simulink model "QueuingSys"  (R2019a)
settings: Solver=VariableStepAuto  StartTime=0.0  StopTime=100  RelTol=1e-3  EnableMultiTasking=on
undefined symbols (not defined in the file or in its folder): m, n
(part 5 of 5)

== matlab function QueuingSys/Distro/MMPPArrivalTime36/MMPP ==
  data: x input; T input; D input; x output; M input; T output; D output; t output; rn input; lambda output
function [x,T,D,t,lambda] = fcn(x,T,D,M,rn)
lambda = sum(M(x,:))-M(x,x);
trn = expinv(rn,lambda);
if trn > T(2)
    D =rand(2,1);
    T2 = expinv(D(2),lambda);
    j = 1;
    a = 0;
    b = sum(M(x,1:j));
    while ~(a < D(1) < b)
        j = j +1;
        a = sum(M(x,1:j));
        b = sum(M(x,1:j));
    end
    x = j;
    T(1) = T(2);
    T(2) = T2;
    lambda = sum(M(x,:))-M(x,x);
    trn = expinv(rn,lambda);
end
% x = j;
t = trn;% x(end);

== matlab function QueuingSys/Distro/MMPPArrivalTime37/MMPP ==
  data: x input; T input; D input; x output; M input; T output; D output; t output; rn input; lambda output
function [x,T,D,t,lambda] = fcn(x,T,D,M,rn)
lambda = sum(M(x,:))-M(x,x);
trn = expinv(rn,lambda);
if trn > T(2)
    D =rand(2,1);
    T2 = expinv(D(2),lambda);
    j = 1;
    a = 0;
    b = sum(M(x,1:j));
    while ~(a < D(1) < b)
        j = j +1;
        a = sum(M(x,1:j));
        b = sum(M(x,1:j));
    end
    x = j;
    T(1) = T(2);
    T(2) = T2;
    lambda = sum(M(x,:))-M(x,x);
    trn = expinv(rn,lambda);
end
% x = j;
t = trn;% x(end);

== matlab function QueuingSys/Distro/MMPPArrivalTime38/MMPP ==
  data: x input; T input; D input; x output; M input; T output; D output; t output; rn input; lambda output
function [x,T,D,t,lambda] = fcn(x,T,D,M,rn)
lambda = sum(M(x,:))-M(x,x);
trn = expinv(rn,lambda);
if trn > T(2)
    D =rand(2,1);
    T2 = expinv(D(2),lambda);
    j = 1;
    a = 0;
    b = sum(M(x,1:j));
    while ~(a < D(1) < b)
        j = j +1;
        a = sum(M(x,1:j));
        b = sum(M(x,1:j));
    end
    x = j;
    T(1) = T(2);
    T(2) = T2;
    lambda = sum(M(x,:))-M(x,x);
    trn = expinv(rn,lambda);
end
% x = j;
t = trn;% x(end);

== matlab function QueuingSys/Distro/MMPPArrivalTime39/MMPP ==
  data: x input; T input; D input; x output; M input; T output; D output; t output; rn input; lambda output
function [x,T,D,t,lambda] = fcn(x,T,D,M,rn)
lambda = sum(M(x,:))-M(x,x);
trn = expinv(rn,lambda);
if trn > T(2)
    D =rand(2,1);
    T2 = expinv(D(2),lambda);
    j = 1;
    a = 0;
    b = sum(M(x,1:j));
    while ~(a < D(1) < b)
        j = j +1;
        a = sum(M(x,1:j));
        b = sum(M(x,1:j));
    end
    x = j;
    T(1) = T(2);
    T(2) = T2;
    lambda = sum(M(x,:))-M(x,x);
    trn = expinv(rn,lambda);
end
% x = j;
t = trn;% x(end);

== matlab function QueuingSys/Distro/MMPPArrivalTime40/MMPP ==
  data: x input; T input; D input; x output; M input; T output; D output; t output; rn input; lambda output
function [x,T,D,t,lambda] = fcn(x,T,D,M,rn)
lambda = sum(M(x,:))-M(x,x);
trn = expinv(rn,lambda);
if trn > T(2)
    D =rand(2,1);
    T2 = expinv(D(2),lambda);
    j = 1;
    a = 0;
    b = sum(M(x,1:j));
    while ~(a < D(1) < b)
        j = j +1;
        a = sum(M(x,1:j));
        b = sum(M(x,1:j));
    end
    x = j;
    T(1) = T(2);
    T(2) = T2;
    lambda = sum(M(x,:))-M(x,x);
    trn = expinv(rn,lambda);
end
% x = j;
t = trn;% x(end);

== matlab function QueuingSys/Distro/MMPPArrivalTime41/MMPP ==
  data: x input; T input; D input; x output; M input; T output; D output; t output; rn input; lambda output
function [x,T,D,t,lambda] = fcn(x,T,D,M,rn)
lambda = sum(M(x,:))-M(x,x);
trn = expinv(rn,lambda);
if trn > T(2)
    D =rand(2,1);
    T2 = expinv(D(2),lambda);
    j = 1;
    a = 0;
    b = sum(M(x,1:j));
    while ~(a < D(1) < b)
        j = j +1;
        a = sum(M(x,1:j));
        b = sum(M(x,1:j));
    end
    x = j;
    T(1) = T(2);
    T(2) = T2;
    lambda = sum(M(x,:))-M(x,x);
    trn = expinv(rn,lambda);
end
% x = j;
t = trn;% x(end);

== matlab function QueuingSys/Distro/MMPPArrivalTime42/MMPP ==
  data: x input; T input; D input; x output; M input; T output; D output; t output; rn input; lambda output
function [x,T,D,t,lambda] = fcn(x,T,D,M,rn)
lambda = sum(M(x,:))-M(x,x);
trn = expinv(rn,lambda);
if trn > T(2)
    D =rand(2,1);
    T2 = expinv(D(2),lambda);
    j = 1;
    a = 0;
    b = sum(M(x,1:j));
    while ~(a < D(1) < b)
        j = j +1;
        a = sum(M(x,1:j));
        b = sum(M(x,1:j));
    end
    x = j;
    T(1) = T(2);
    T(2) = T2;
    lambda = sum(M(x,:))-M(x,x);
    trn = expinv(rn,lambda);
end
% x = j;
t = trn;% x(end);

== matlab function QueuingSys/Distro/MMPPArrivalTime43/MMPP ==
  data: x input; T input; D input; x output; M input; T output; D output; t output; rn input; lambda output
function [x,T,D,t,lambda] = fcn(x,T,D,M,rn)
lambda = sum(M(x,:))-M(x,x);
trn = expinv(rn,lambda);
if trn > T(2)
    D =rand(2,1);
    T2 = expinv(D(2),lambda);
    j = 1;
    a = 0;
    b = sum(M(x,1:j));
    while ~(a < D(1) < b)
        j = j +1;
        a = sum(M(x,1:j));
        b = sum(M(x,1:j));
    end
    x = j;
    T(1) = T(2);
    T(2) = T2;
    lambda = sum(M(x,:))-M(x,x);
    trn = expinv(rn,lambda);
end
% x = j;
t = trn;% x(end);

== matlab function QueuingSys/Distro/MMPPArrivalTime44/MMPP ==
  data: x input; T input; D input; x output; M input; T output; D output; t output; rn input; lambda output
function [x,T,D,t,lambda] = fcn(x,T,D,M,rn)
lambda = sum(M(x,:))-M(x,x);
trn = expinv(rn,lambda);
if trn > T(2)
    D =rand(2,1);
    T2 = expinv(D(2),lambda);
    j = 1;
    a = 0;
    b = sum(M(x,1:j));
    while ~(a < D(1) < b)
        j = j +1;
        a = sum(M(x,1:j));
        b = sum(M(x,1:j));
    end
    x = j;
    T(1) = T(2);
    T(2) = T2;
    lambda = sum(M(x,:))-M(x,x);
    trn = expinv(rn,lambda);
end
% x = j;
t = trn;% x(end);

== matlab function QueuingSys/Distro/MMPPArrivalTime45/MMPP ==
  data: x input; T input; D input; x output; M input; T output; D output; t output; rn input; lambda output
function [x,T,D,t,lambda] = fcn(x,T,D,M,rn)
lambda = sum(M(x,:))-M(x,x);
trn = expinv(rn,lambda);
if trn > T(2)
    D =rand(2,1);
    T2 = expinv(D(2),lambda);
    j = 1;
    a = 0;
    b = sum(M(x,1:j));
    while ~(a < D(1) < b)
        j = j +1;
        a = sum(M(x,1:j));
        b = sum(M(x,1:j));
    end
    x = j;
    T(1) = T(2);
    T(2) = T2;
    lambda = sum(M(x,:))-M(x,x);
    trn = expinv(rn,lambda);
end
% x = j;
t = trn;% x(end);

== matlab function QueuingSys/Distro/MMPPArrivalTime46/MMPP ==
  data: x input; T input; D input; x output; M input; T output; D output; t output; rn input; lambda output
function [x,T,D,t,lambda] = fcn(x,T,D,M,rn)
lambda = sum(M(x,:))-M(x,x);
trn = expinv(rn,lambda);
if trn > T(2)
    D =rand(2,1);
    T2 = expinv(D(2),lambda);
    j = 1;
    a = 0;
    b = sum(M(x,1:j));
    while ~(a < D(1) < b)
        j = j +1;
        a = sum(M(x,1:j));
        b = sum(M(x,1:j));
    end
    x = j;
    T(1) = T(2);
    T(2) = T2;
    lambda = sum(M(x,:))-M(x,x);
    trn = expinv(rn,lambda);
end
% x = j;
t = trn;% x(end);

== matlab function QueuingSys/Distro/MMPPArrivalTime47/MMPP ==
  data: x input; T input; D input; x output; M input; T output; D output; t output; rn input; lambda output
function [x,T,D,t,lambda] = fcn(x,T,D,M,rn)
lambda = sum(M(x,:))-M(x,x);
trn = expinv(rn,lambda);
if trn > T(2)
    D =rand(2,1);
    T2 = expinv(D(2),lambda);
    j = 1;
    a = 0;
    b = sum(M(x,1:j));
    while ~(a < D(1) < b)
        j = j +1;
        a = sum(M(x,1:j));
        b = sum(M(x,1:j));
    end
    x = j;
    T(1) = T(2);
    T(2) = T2;
    lambda = sum(M(x,:))-M(x,x);
    trn = expinv(rn,lambda);
end
% x = j;
t = trn;% x(end);

== matlab function QueuingSys/Distro/MMPPArrivalTime48/MMPP ==
  data: x input; T input; D input; x output; M input; T output; D output; t output; rn input; lambda output
function [x,T,D,t,lambda] = fcn(x,T,D,M,rn)
lambda = sum(M(x,:))-M(x,x);
trn = expinv(rn,lambda);
if trn > T(2)
    D =rand(2,1);
    T2 = expinv(D(2),lambda);
    j = 1;
    a = 0;
    b = sum(M(x,1:j));
    while ~(a < D(1) < b)
        j = j +1;
        a = sum(M(x,1:j));
        b = sum(M(x,1:j));
    end
    x = j;
    T(1) = T(2);
    T(2) = T2;
    lambda = sum(M(x,:))-M(x,x);
    trn = expinv(rn,lambda);
end
% x = j;
t = trn;% x(end);

== matlab function QueuingSys/Distro/MMPPArrivalTime49/MMPP ==
  data: x input; T input; D input; x output; M input; T output; D output; t output; rn input; lambda output
function [x,T,D,t,lambda] = fcn(x,T,D,M,rn)
lambda = sum(M(x,:))-M(x,x);
trn = expinv(rn,lambda);
if trn > T(2)
    D =rand(2,1);
    T2 = expinv(D(2),lambda);
    j = 1;
    a = 0;
    b = sum(M(x,1:j));
    while ~(a < D(1) < b)
        j = j +1;
        a = sum(M(x,1:j));
        b = sum(M(x,1:j));
    end
    x = j;
    T(1) = T(2);
    T(2) = T2;
    lambda = sum(M(x,:))-M(x,x);
    trn = expinv(rn,lambda);
end
% x = j;
t = trn;% x(end);

== matlab function QueuingSys/Distro/MMPPArrivalTime50/MMPP ==
  data: x input; T input; D input; x output; M input; T output; D output; t output; rn input; lambda output
function [x,T,D,t,lambda] = fcn(x,T,D,M,rn)
lambda = sum(M(x,:))-M(x,x);
trn = expinv(rn,lambda);
if trn > T(2)
    D =rand(2,1);
    T2 = expinv(D(2),lambda);
    j = 1;
    a = 0;
    b = sum(M(x,1:j));
    while ~(a < D(1) < b)
        j = j +1;
        a = sum(M(x,1:j));
        b = sum(M(x,1:j));
    end
    x = j;
    T(1) = T(2);
    T(2) = T2;
    lambda = sum(M(x,:))-M(x,x);
    trn = expinv(rn,lambda);
end
% x = j;
t = trn;% x(end);

== matlab function QueuingSys/Distro/MMPPArrivalTime51/MMPP ==
  data: x input; T input; D input; x output; M input; T output; D output; t output; rn input; lambda output
function [x,T,D,t,lambda] = fcn(x,T,D,M,rn)
lambda = sum(M(x,:))-M(x,x);
trn = expinv(rn,lambda);
if trn > T(2)
    D =rand(2,1);
    T2 = expinv(D(2),lambda);
    j = 1;
    a = 0;
    b = sum(M(x,1:j));
    while ~(a < D(1) < b)
        j = j +1;
        a = sum(M(x,1:j));
        b = sum(M(x,1:j));
    end
    x = j;
    T(1) = T(2);
    T(2) = T2;
    lambda = sum(M(x,:))-M(x,x);
    trn = expinv(rn,lambda);
end
% x = j;
t = trn;% x(end);

== matlab function QueuingSys/Distro/MMPPArrivalTime52/MMPP ==
  data: x input; T input; D input; x output; M input; T output; D output; t output; rn input; lambda output
function [x,T,D,t,lambda] = fcn(x,T,D,M,rn)
lambda = sum(M(x,:))-M(x,x);
trn = expinv(rn,lambda);
if trn > T(2)
    D =rand(2,1);
    T2 = expinv(D(2),lambda);
    j = 1;
    a = 0;
    b = sum(M(x,1:j));
    while ~(a < D(1) < b)
        j = j +1;
        a = sum(M(x,1:j));
        b = sum(M(x,1:j));
    end
    x = j;
    T(1) = T(2);
    T(2) = T2;
    lambda = sum(M(x,:))-M(x,x);
    trn = expinv(rn,lambda);
end
% x = j;
t = trn;% x(end);

== matlab function QueuingSys/Distro/MMPPArrivalTime53/MMPP ==
  data: x input; T input; D input; x output; M input; T output; D output; t output; rn input; lambda output
function [x,T,D,t,lambda] = fcn(x,T,D,M,rn)
lambda = sum(M(x,:))-M(x,x);
trn = expinv(rn,lambda);
if trn > T(2)
    D =rand(2,1);
    T2 = expinv(D(2),lambda);
    j = 1;
    a = 0;
    b = sum(M(x,1:j));
    while ~(a < D(1) < b)
        j = j +1;
        a = sum(M(x,1:j));
        b = sum(M(x,1:j));
    end
    x = j;
    T(1) = T(2);
    T(2) = T2;
    lambda = sum(M(x,:))-M(x,x);
    trn = expinv(rn,lambda);
end
% x = j;
t = trn;% x(end);

== matlab function QueuingSys/Distro/MMPPArrivalTime54/MMPP ==
  data: x input; T input; D input; x output; M input; T output; D output; t output; rn input; lambda output
function [x,T,D,t,lambda] = fcn(x,T,D,M,rn)
lambda = sum(M(x,:))-M(x,x);
trn = expinv(rn,lambda);
if trn > T(2)
    D =rand(2,1);
    T2 = expinv(D(2),lambda);
    j = 1;
    a = 0;
    b = sum(M(x,1:j));
    while ~(a < D(1) < b)
        j = j +1;
        a = sum(M(x,1:j));
        b = sum(M(x,1:j));
    end
    x = j;
    T(1) = T(2);
    T(2) = T2;
    lambda = sum(M(x,:))-M(x,x);
    trn = expinv(rn,lambda);
end
% x = j;
t = trn;% x(end);

== matlab function QueuingSys/Distro/MMPPArrivalTime55/MMPP ==
  data: x input; T input; D input; x output; M input; T output; D output; t output; rn input; lambda output
function [x,T,D,t,lambda] = fcn(x,T,D,M,rn)
lambda = sum(M(x,:))-M(x,x);
trn = expinv(rn,lambda);
if trn > T(2)
    D =rand(2,1);
    T2 = expinv(D(2),lambda);
    j = 1;
    a = 0;
    b = sum(M(x,1:j));
    while ~(a < D(1) < b)
        j = j +1;
        a = sum(M(x,1:j));
        b = sum(M(x,1:j));
    end
    x = j;
    T(1) = T(2);
    T(2) = T2;
    lambda = sum(M(x,:))-M(x,x);
    trn = expinv(rn,lambda);
end
% x = j;
t = trn;% x(end);

== matlab function QueuingSys/Distro/MMPPArrivalTime56/MMPP ==
  data: x input; T input; D input; x output; M input; T output; D output; t output; rn input; lambda output
function [x,T,D,t,lambda] = fcn(x,T,D,M,rn)
lambda = sum(M(x,:))-M(x,x);
trn = expinv(rn,lambda);
if trn > T(2)
    D =rand(2,1);
    T2 = expinv(D(2),lambda);
    j = 1;
    a = 0;
    b = sum(M(x,1:j));
    while ~(a < D(1) < b)
        j = j +1;
        a = sum(M(x,1:j));
        b = sum(M(x,1:j));
    end
    x = j;
    T(1) = T(2);
    T(2) = T2;
    lambda = sum(M(x,:))-M(x,x);
    trn = expinv(rn,lambda);
end
% x = j;
t = trn;% x(end);

== matlab function QueuingSys/Distro/MMPPArrivalTime57/MMPP ==
  data: x input; T input; D input; x output; M input; T output; D output; t output; rn input; lambda output
function [x,T,D,t,lambda] = fcn(x,T,D,M,rn)
lambda = sum(M(x,:))-M(x,x);
trn = expinv(rn,lambda);
if trn > T(2)
    D =rand(2,1);
    T2 = expinv(D(2),lambda);
    j = 1;
    a = 0;
    b = sum(M(x,1:j));
    while ~(a < D(1) < b)
        j = j +1;
        a = sum(M(x,1:j));
        b = sum(M(x,1:j));
    end
    x = j;
    T(1) = T(2);
    T(2) = T2;
    lambda = sum(M(x,:))-M(x,x);
    trn = expinv(rn,lambda);
end
% x = j;
t = trn;% x(end);

== matlab function QueuingSys/Distro/MMPPArrivalTime58/MMPP ==
  data: x input; T input; D input; x output; M input; T output; D output; t output; rn input; lambda output
function [x,T,D,t,lambda] = fcn(x,T,D,M,rn)
lambda = sum(M(x,:))-M(x,x);
trn = expinv(rn,lambda);
if trn > T(2)
    D =rand(2,1);
    T2 = expinv(D(2),lambda);
    j = 1;
    a = 0;
    b = sum(M(x,1:j));
    while ~(a < D(1) < b)
        j = j +1;
        a = sum(M(x,1:j));
        b = sum(M(x,1:j));
    end
    x = j;
    T(1) = T(2);
    T(2) = T2;
    lambda = sum(M(x,:))-M(x,x);
    trn = expinv(rn,lambda);
end
% x = j;
t = trn;% x(end);

== matlab function QueuingSys/Distro/MMPPArrivalTime59/MMPP ==
  data: x input; T input; D input; x output; M input; T output; D output; t output; rn input; lambda output
function [x,T,D,t,lambda] = fcn(x,T,D,M,rn)
lambda = sum(M(x,:))-M(x,x);
trn = expinv(rn,lambda);
if trn > T(2)
    D =rand(2,1);
    T2 = expinv(D(2),lambda);
    j = 1;
    a = 0;
    b = sum(M(x,1:j));
    while ~(a < D(1) < b)
        j = j +1;
        a = sum(M(x,1:j));
        b = sum(M(x,1:j));
    end
    x = j;
    T(1) = T(2);
    T(2) = T2;
    lambda = sum(M(x,:))-M(x,x);
    trn = expinv(rn,lambda);
end
% x = j;
t = trn;% x(end);

== matlab function QueuingSys/Distro/MMPPArrivalTime60/MMPP ==
  data: x input; T input; D input; x output; M input; T output; D output; t output; rn input; lambda output
function [x,T,D,t,lambda] = fcn(x,T,D,M,rn)
lambda = sum(M(x,:))-M(x,x);
trn = expinv(rn,lambda);
if trn > T(2)
    D =rand(2,1);
    T2 = expinv(D(2),lambda);
    j = 1;
    a = 0;
    b = sum(M(x,1:j));
    while ~(a < D(1) < b)
        j = j +1;
        a = sum(M(x,1:j));
        b = sum(M(x,1:j));
    end
    x = j;
    T(1) = T(2);
    T(2) = T2;
    lambda = sum(M(x,:))-M(x,x);
    trn = expinv(rn,lambda);
end
% x = j;
t = trn;% x(end);

== matlab function QueuingSys/Distro/MMPPArrivalTime61/MMPP ==
  data: x input; T input; D input; x output; M input; T output; D output; t output; rn input; lambda output
function [x,T,D,t,lambda] = fcn(x,T,D,M,rn)
lambda = sum(M(x,:))-M(x,x);
trn = expinv(rn,lambda);
if trn > T(2)
    D =rand(2,1);
    T2 = expinv(D(2),lambda);
    j = 1;
    a = 0;
    b = sum(M(x,1:j));
    while ~(a < D(1) < b)
        j = j +1;
        a = sum(M(x,1:j));
        b = sum(M(x,1:j));
    end
    x = j;
    T(1) = T(2);
    T(2) = T2;
    lambda = sum(M(x,:))-M(x,x);
    trn = expinv(rn,lambda);
end
% x = j;
t = trn;% x(end);

== matlab function QueuingSys/Distro/MMPPArrivalTime62/MMPP ==
  data: x input; T input; D input; x output; M input; T output; D output; t output; rn input; lambda output
function [x,T,D,t,lambda] = fcn(x,T,D,M,rn)
lambda = sum(M(x,:))-M(x,x);
trn = expinv(rn,lambda);
if trn > T(2)
    D =rand(2,1);
    T2 = expinv(D(2),lambda);
    j = 1;
    a = 0;
    b = sum(M(x,1:j));
    while ~(a < D(1) < b)
        j = j +1;
        a = sum(M(x,1:j));
        b = sum(M(x,1:j));
    end
    x = j;
    T(1) = T(2);
    T(2) = T2;
    lambda = sum(M(x,:))-M(x,x);
    trn = expinv(rn,lambda);
end
% x = j;
t = trn;% x(end);

== matlab function QueuingSys/Distro/MMPPArrivalTime63/MMPP ==
  data: x input; T input; D input; x output; M input; T output; D output; t output; rn input; lambda output
function [x,T,D,t,lambda] = fcn(x,T,D,M,rn)
lambda = sum(M(x,:))-M(x,x);
trn = expinv(rn,lambda);
if trn > T(2)
    D =rand(2,1);
    T2 = expinv(D(2),lambda);
    j = 1;
    a = 0;
    b = sum(M(x,1:j));
    while ~(a < D(1) < b)
        j = j +1;
        a = sum(M(x,1:j));
        b = sum(M(x,1:j));
    end
    x = j;
    T(1) = T(2);
    T(2) = T2;
    lambda = sum(M(x,:))-M(x,x);
    trn = expinv(rn,lambda);
end
% x = j;
t = trn;% x(end);

== matlab function QueuingSys/Distro/MMPPArrivalTime64/MMPP ==
  data: x input; T input; D input; x output; M input; T output; D output; t output; rn input; lambda output
function [x,T,D,t,lambda] = fcn(x,T,D,M,rn)
lambda = sum(M(x,:))-M(x,x);
trn = expinv(rn,lambda);
if trn > T(2)
    D =rand(2,1);
    T2 = expinv(D(2),lambda);
    j = 1;
    a = 0;
    b = sum(M(x,1:j));
    while ~(a < D(1) < b)
        j = j +1;
        a = sum(M(x,1:j));
        b = sum(M(x,1:j));
    end
    x = j;
    T(1) = T(2);
    T(2) = T2;
    lambda = sum(M(x,:))-M(x,x);
    trn = expinv(rn,lambda);
end
% x = j;
t = trn;% x(end);

== matlab function QueuingSys/Distro/MMPPArrivalTime65/MMPP ==
  data: x input; T input; D input; x output; M input; T output; D output; t output; rn input; lambda output
function [x,T,D,t,lambda] = fcn(x,T,D,M,rn)
lambda = sum(M(x,:))-M(x,x);
trn = expinv(rn,lambda);
if trn > T(2)
    D =rand(2,1);
    T2 = expinv(D(2),lambda);
    j = 1;
    a = 0;
    b = sum(M(x,1:j));
    while ~(a < D(1) < b)
        j = j +1;
        a = sum(M(x,1:j));
        b = sum(M(x,1:j));
    end
    x = j;
    T(1) = T(2);
    T(2) = T2;
    lambda = sum(M(x,:))-M(x,x);
    trn = expinv(rn,lambda);
end
% x = j;
t = trn;% x(end);

== matlab function QueuingSys/Distro/MMPPArrivalTime66/MMPP ==
  data: x input; T input; D input; x output; M input; T output; D output; t output; rn input; lambda output
function [x,T,D,t,lambda] = fcn(x,T,D,M,rn)
lambda = sum(M(x,:))-M(x,x);
trn = expinv(rn,lambda);
if trn > T(2)
    D =rand(2,1);
    T2 = expinv(D(2),lambda);
    j = 1;
    a = 0;
    b = sum(M(x,1:j));
    while ~(a < D(1) < b)
        j = j +1;
        a = sum(M(x,1:j));
        b = sum(M(x,1:j));
    end
    x = j;
    T(1) = T(2);
    T(2) = T2;
    lambda = sum(M(x,:))-M(x,x);
    trn = expinv(rn,lambda);
end
% x = j;
t = trn;% x(end);

== matlab function QueuingSys/Distro/MMPPArrivalTime67/MMPP ==
  data: x input; T input; D input; x output; M input; T output; D output; t output; rn input; lambda output
function [x,T,D,t,lambda] = fcn(x,T,D,M,rn)
lambda = sum(M(x,:))-M(x,x);
trn = expinv(rn,lambda);
if trn > T(2)
    D =rand(2,1);
    T2 = expinv(D(2),lambda);
    j = 1;
    a = 0;
    b = sum(M(x,1:j));
    while ~(a < D(1) < b)
        j = j +1;
        a = sum(M(x,1:j));
        b = sum(M(x,1:j));
    end
    x = j;
    T(1) = T(2);
    T(2) = T2;
    lambda = sum(M(x,:))-M(x,x);
    trn = expinv(rn,lambda);
end
% x = j;
t = trn;% x(end);

== matlab function QueuingSys/Distro/MMPPArrivalTime68/MMPP ==
  data: x input; T input; D input; x output; M input; T output; D output; t output; rn input; lambda output
function [x,T,D,t,lambda] = fcn(x,T,D,M,rn)
lambda = sum(M(x,:))-M(x,x);
trn = expinv(rn,lambda);
if trn > T(2)
    D =rand(2,1);
    T2 = expinv(D(2),lambda);
    j = 1;
    a = 0;
    b = sum(M(x,1:j));
    while ~(a < D(1) < b)
        j = j +1;
        a = sum(M(x,1:j));
        b = sum(M(x,1:j));
    end
    x = j;
    T(1) = T(2);
    T(2) = T2;
    lambda = sum(M(x,:))-M(x,x);
    trn = expinv(rn,lambda);
end
% x = j;
t = trn;% x(end);

== matlab function QueuingSys/Distro/MMPPArrivalTime69/MMPP ==
  data: x input; T input; D input; x output; M input; T output; D output; t output; rn input; lambda output
function [x,T,D,t,lambda] = fcn(x,T,D,M,rn)
lambda = sum(M(x,:))-M(x,x);
trn = expinv(rn,lambda);
if trn > T(2)
    D =rand(2,1);
    T2 = expinv(D(2),lambda);
    j = 1;
    a = 0;
    b = sum(M(x,1:j));
    while ~(a < D(1) < b)
        j = j +1;
        a = sum(M(x,1:j));
        b = sum(M(x,1:j));
    end
    x = j;
    T(1) = T(2);
    T(2) = T2;
    lambda = sum(M(x,:))-M(x,x);
    trn = expinv(rn,lambda);
end
% x = j;
t = trn;% x(end);

== matlab function QueuingSys/Distro/MMPPArrivalTime70/MMPP ==
  data: x input; T input; D input; x output; M input; T output; D output; t output; rn input; lambda output
function [x,T,D,t,lambda] = fcn(x,T,D,M,rn)
lambda = sum(M(x,:))-M(x,x);
trn = expinv(rn,lambda);
if trn > T(2)
    D =rand(2,1);
    T2 = expinv(D(2),lambda);
    j = 1;
    a = 0;
    b = sum(M(x,1:j));
    while ~(a < D(1) < b)
        j = j +1;
        a = sum(M(x,1:j));
        b = sum(M(x,1:j));
    end
    x = j;
    T(1) = T(2);
    T(2) = T2;
    lambda = sum(M(x,:))-M(x,x);
    trn = expinv(rn,lambda);
end
% x = j;
t = trn;% x(end);
